simulink model "load8"  (Simulink 8.5)
settings: Solver=ode15s  SolverMode=SingleTasking  StartTime=0.0  StopTime=0.1  RelTol=1e-3  AbsTol=1e-6
libraries: powerlib x27
settings Model: Creator=Dr. Lotfifard  LastModifiedBy=PC
settings DataIOCC: LimitDataPoints=off
settings OptimizationCC: BlockReduction=off  BooleanDataType=off
settings DebuggingCC: SaveWithParameterizedLinksMsg=none  SignalResolutionControl=TryResolveAllWithWarning  MultiTaskDSMMsg=warning  MultiTaskCondExecSysMsg=none  FcnCallInpInsideContextMsg=UseLocalSettings  StrictBusMsg=None
settings HardwareCC: TargetUnknown=on

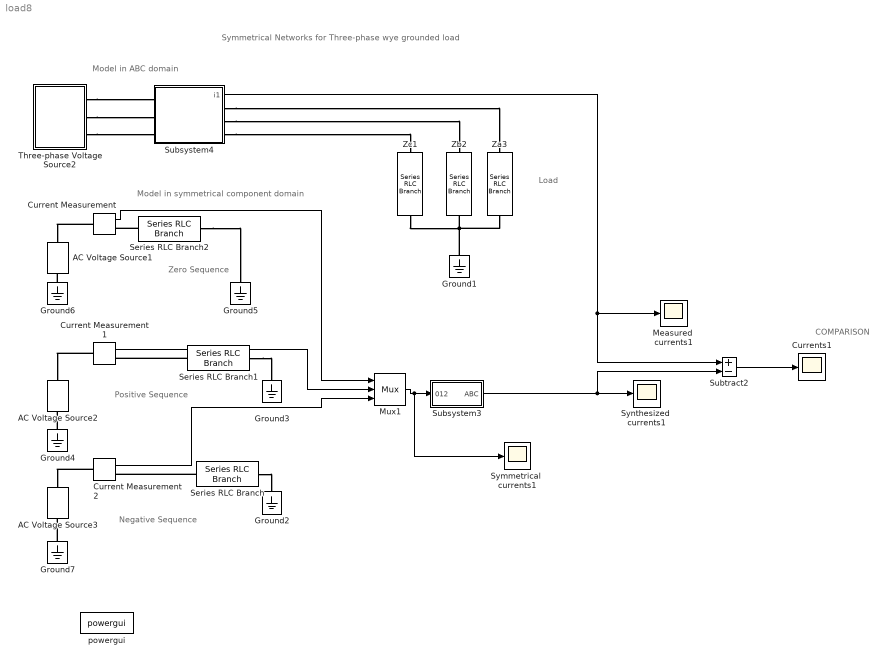
== system load8 ==
  note: Symmetrical Networks for Three-phase wye grounded load
  note: Model in ABC domain
  note: Model in symmetrical component domain
  note: COMPARISON
  note: Zero
      | Sequence
  note: Positive
      | Sequence
  note: Negative
      | Sequence
  note: Load
  " Currents1" : Scope
      settings: TickLabels=on  TimeRange=0.1  YMin=-3  YMax=3
  AC Voltage Source1 : powerlib/Electrical Sources/AC Voltage Source  Amplitude=0.031  Phase=-78  Frequency=60  SampleTime=0  Measurements=None
  AC Voltage Source2 : powerlib/Electrical Sources/AC Voltage Source  Amplitude=0.963  Phase=-6.56  Frequency=60  SampleTime=0  Measurements=None
  AC Voltage Source3 : powerlib/Electrical Sources/AC Voltage Source  Amplitude=0.145  Phase=75.41  Frequency=60  SampleTime=0  Measurements=None
  Current Measurement : powerlib/Measurements/Current Measurement  PhasorSimulation=off  OutputType=Complex  PSBequivalent=0
  Current Measurement1 : powerlib/Measurements/Current Measurement  PhasorSimulation=off  OutputType=Complex  PSBequivalent=0
  Current Measurement2 : powerlib/Measurements/Current Measurement  PhasorSimulation=off  OutputType=Complex  PSBequivalent=0
  Ground{1..7} (7 alike) : powerlib/Elements/Ground  LConnTagsString=a
  Measured  currents1 : Scope
      settings: TickLabels=on  TimeRange=0.1
  Mux1 : Mux  Inputs=3
  Series RLC Branch : powerlib/Elements/Series RLC Branch  LConnTagsString=__new0  RConnTagsString=__new0  BranchType=RL  Resistance=1  Inductance=1e-3  SetiL0=off  InitialCurrent=0  Capacitance=1e-6  Setx0=off  InitialVoltage=0  Measurements=None
  Series RLC Branch1 : powerlib/Elements/Series RLC Branch  LConnTagsString=__new0  RConnTagsString=__new0  BranchType=RL  Resistance=1  Inductance=1e-3  SetiL0=off  InitialCurrent=0  Capacitance=1e-6  Setx0=off  InitialVoltage=0  Measurements=None
  Series RLC Branch2 : powerlib/Elements/Series RLC Branch  LConnTagsString=__new0  RConnTagsString=__new0  BranchType=RL  Resistance=1  Inductance=1e-3  SetiL0=off  InitialCurrent=0  Capacitance=1e-6  Setx0=off  InitialVoltage=0  Measurements=None
  Subsystem3 : Subsystem
  Subsystem4 : Subsystem
      mask Display: disp('Current\nMeasurements')
  Subtract2 : Sum  Inputs=+-  SaturateOnIntegerOverflow=on  InputSameDT=on  OutDataTypeStr=Inherit: Same as first input
  Symmetrical  currents1 : Scope
      settings: TickLabels=on  TimeRange=0.1  SaveName=ScopeData2
  Synthesized  currents1 : Scope
      settings: TickLabels=on  TimeRange=0.1  SaveName=ScopeData3
  Three-phase Voltage Source2 : Subsystem
  Za3 : powerlib/Elements/Series RLC Branch  LConnTagsString=__new0  RConnTagsString=__new0  BranchType=RL  Resistance=0.1  Inductance=0.3/(2*pi*60)  SetiL0=off  InitialCurrent=0  Capacitance=1e-6  Setx0=off  InitialVoltage=0  Measurements=None
  Zb2 : powerlib/Elements/Series RLC Branch  LConnTagsString=__new0  RConnTagsString=__new0  BranchType=RL  Resistance=0.1  Inductance=0.4/(2*pi*60)  SetiL0=off  InitialCurrent=0  Capacitance=1e-6  Setx0=off  InitialVoltage=0  Measurements=None
  Zc1 : powerlib/Elements/Series RLC Branch  LConnTagsString=__new0  RConnTagsString=__new0  BranchType=RL  Resistance=0.1  Inductance=0.4/(2*pi*60)  SetiL0=off  InitialCurrent=0  Capacitance=1e-6  Setx0=off  InitialVoltage=0  Measurements=None
  powergui : powerlib/powergui  SimulationMode=Continuous  SolverType=Tustin/Backward Euler (TBE)  SampleTime=0  frequency=60  SPID=off  DisableSnubberDevices=off  DisableRonSwitches=off  DisableVfSwitches=off  SwTol=0  DisplayEquations=off  Interpol=off  methode=off  Ts=0  FunctionMessages=off  echomessages=off  HookPort=off  EnableUseOfTLC=off  x0status=blocks  frequencyindice=60  Pbase=100e6  ErrMax=1e-4  Iterations=50  UnitsV=kV  UnitsW=MW  buscounter=0  RestoreLinks=warning  ResistiveCurrentMeasurement=off  Frange=[0:2:500]  Ylog=off  Xlog=on  ShowGrid=off  save=off  variable=ZData  structure=0  ZoomFFT=on  StartTime=0.0  cycles=1  DisplayStyle=1  fundamental=60  FreqAxis=off  MaxFrequency=1000  frequencyindicesteady=1  RmsSteady=1  display=off
  wires:
  Mux1/1 -> Subsystem3/1(012), Symmetrical  currents1/1
  Subtract2/1 -> " Currents1"/1
  Subsystem3/1(ABC) -> Synthesized  currents1/1, Subtract2/2
  Subsystem4/1(i1) -> Measured  currents1/1, Subtract2/1
  Current Measurement2/1 -> Mux1/3
  Current Measurement1/1 -> Mux1/2
  Current Measurement/1 -> Mux1/1
  connections:
  Ground6/LConn1 -- AC Voltage Source1/LConn1
  Ground1/LConn1 -- Za3/RConn1 -- Zc1/RConn1 -- Zb2/RConn1
  Ground7/LConn1 -- AC Voltage Source3/LConn1
  Three-phase Voltage Source2/RConn3 -- Subsystem4/LConn3
  Subsystem4/RConn1 -- Za3/LConn1
  Ground4/LConn1 -- AC Voltage Source2/LConn1
  Current Measurement1/LConn1 -- AC Voltage Source2/RConn1
  Current Measurement2/LConn1 -- AC Voltage Source3/RConn1
  Series RLC Branch1/RConn1 -- Ground3/LConn1
  Subsystem4/RConn2 -- Zb2/LConn1
  Series RLC Branch/LConn1 -- Current Measurement2/RConn1
  Current Measurement/LConn1 -- AC Voltage Source1/RConn1
  Series RLC Branch/RConn1 -- Ground2/LConn1
  Three-phase Voltage Source2/RConn1 -- Subsystem4/LConn1
  Series RLC Branch2/LConn1 -- Current Measurement/RConn1
  Three-phase Voltage Source2/RConn2 -- Subsystem4/LConn2
  Series RLC Branch1/LConn1 -- Current Measurement1/RConn1
  Subsystem4/RConn3 -- Zc1/LConn1
  Series RLC Branch2/RConn1 -- Ground5/LConn1

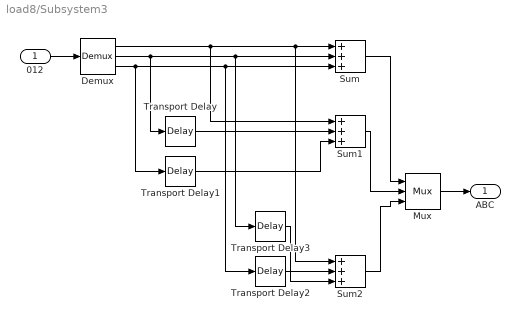
== system load8/Subsystem3 ==
  012 : Inport
  Demux : Demux  Outputs=3
  Mux : Mux  Inputs=3
  Sum : Sum  Inputs=+++  SaturateOnIntegerOverflow=on  InputSameDT=on  OutDataTypeStr=Inherit: Same as first input
  Sum1 : Sum  Inputs=+++  SaturateOnIntegerOverflow=on  InputSameDT=on  OutDataTypeStr=Inherit: Same as first input
  Sum2 : Sum  Inputs=+++  SaturateOnIntegerOverflow=on  InputSameDT=on  OutDataTypeStr=Inherit: Same as first input
  Transport Delay : TransportDelay  DelayTime=1/(3*60)
  Transport Delay1 : TransportDelay  DelayTime=2/(3*60)
  Transport Delay2 : TransportDelay  DelayTime=1/(3*60)
  Transport Delay3 : TransportDelay  DelayTime=2/(3*60)
  ABC : Outport  InitialOutput=0
  wires:
  012/1 -> Demux/1
  Sum1/1 -> Mux/2
  Sum/1 -> Mux/1
  Mux/1 -> ABC/1
  Sum2/1 -> Mux/3
  Demux/2 -> Transport Delay/1, Sum/2, Transport Delay3/1
  Demux/3 -> Transport Delay1/1, Sum/3, Transport Delay2/1
  Demux/1 -> Sum1/1, Sum/1, Sum2/1
  Transport Delay/1 -> Sum1/2
  Transport Delay1/1 -> Sum1/3
  Transport Delay2/1 -> Sum2/3
  Transport Delay3/1 -> Sum2/2

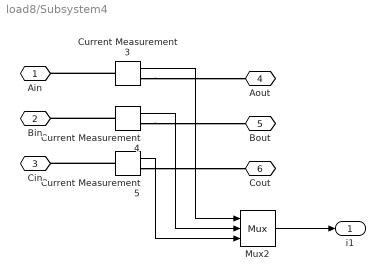
== system load8/Subsystem4 ==
  Current Measurement3 : powerlib/Measurements/Current Measurement  PhasorSimulation=off  OutputType=Complex  PSBequivalent=0
  Current Measurement4 : powerlib/Measurements/Current Measurement  PhasorSimulation=off  OutputType=Complex  PSBequivalent=0
  Current Measurement5 : powerlib/Measurements/Current Measurement  PhasorSimulation=off  OutputType=Complex  PSBequivalent=0
  Mux2 : Mux  Inputs=3
  Ain : PMIOPort  Port=1  Side=Left
  Bin : PMIOPort  Port=2  Side=Left
  Cin : PMIOPort  Port=3  Side=Left
  Aout : PMIOPort  Port=4  Side=Right
  Bout : PMIOPort  Port=5  Side=Right
  Cout : PMIOPort  Port=6  Side=Right
  i1 : Outport  InitialOutput=0
  wires:
  Current Measurement3/1 -> Mux2/1
  Current Measurement4/1 -> Mux2/2
  Current Measurement5/1 -> Mux2/3
  Mux2/1 -> i1/1
  connections:
  Current Measurement3/LConn1 -- Ain/RConn1
  Current Measurement4/LConn1 -- Bin/RConn1
  Current Measurement5/LConn1 -- Cin/RConn1
  Current Measurement3/RConn1 -- Aout/RConn1
  Current Measurement4/RConn1 -- Bout/RConn1
  Current Measurement5/RConn1 -- Cout/RConn1

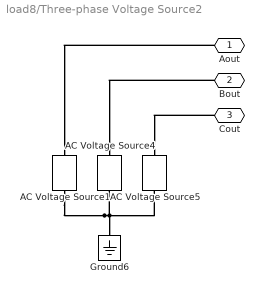
== system load8/Three-phase Voltage Source2 ==
  AC Voltage Source1 : powerlib/Electrical Sources/AC Voltage Source  Amplitude=1  Phase=0  Frequency=60  SampleTime=0  Measurements=None
  AC Voltage Source4 : powerlib/Electrical Sources/AC Voltage Source  Amplitude=1.1  Phase=-130  Frequency=60  SampleTime=0  Measurements=None
  AC Voltage Source5 : powerlib/Electrical Sources/AC Voltage Source  Amplitude=0.8  Phase=110  Frequency=60  SampleTime=0  Measurements=None
  Ground6 : powerlib/Elements/Ground  LConnTagsString=a
  Aout : PMIOPort  Port=1  Side=Right
  Bout : PMIOPort  Port=2  Side=Right
  Cout : PMIOPort  Port=3  Side=Right
  connections:
  AC Voltage Source5/LConn1 -- AC Voltage Source1/LConn1 -- Ground6/LConn1 -- AC Voltage Source4/LConn1
  Cout/RConn1 -- AC Voltage Source5/RConn1
  Bout/RConn1 -- AC Voltage Source4/RConn1
  Aout/RConn1 -- AC Voltage Source1/RConn1
